simulink model "smueqq"  (R2017a)
settings: Solver=VariableStepAuto  StartTime=0.0  StopTime=180  RelTol=1e-3
libraries: dsparch4 x5, simulink x5, dspsnks4 x1, dspvision x1
settings Model: Creator=achar  LastModifiedBy=achar

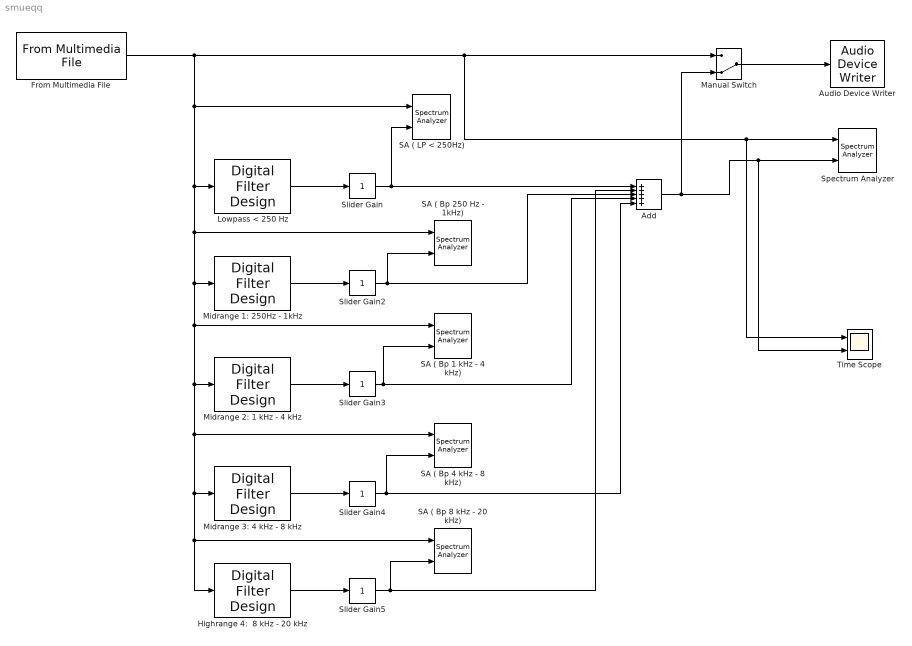
== system smueqq ==
  " Lowpass < 250 Hz " : dsparch4/Digital Filter Design  mwdsp_browser_bugfix_var=off
  Add : Sum  Inputs=+++++
  Audio Device Writer : dspsnks4/Audio Device Writer  Driver=DirectSound  Device=Default  InheritSampleRate=on  SampleRate=44100  BitDepth=16-bit integer  BufferSize=4096  NumBuffers=10  DefaultOutputChannelMapping=on  OutputChannelMapping=1:2  OutputNumUnderrunSamples=off  DriverIdx=1  DeviceWarnFlag=''
  From Multimedia File : dspvision/From Multimedia File  inputFilename=D:\BitBucketLocalRepository\projects\digital_signal_processing\P1_5_band_Audio_Equalizer_Matlab\FIR_BASED\BE_OE.mp3  loop=on  numPlays=inf  outputStreams=Audio only  videoDataType=single  audioDataType=double  inheritSampleTime=on  userDefinedSampleTime=1/30  noAudioOutput=off  isIntensityVideo=off  fourcc=RGB  colorVideoFormat=Separate color signals  outputEOF=off  dataOrg=Column-major  audioFrameSize=1024  computeAudioFrameSize=off  outSamplingMode=Sample based
      settings: SourceProductBaseCode=VP
  Highrange 4:  8 kHz - 20 kHz : dsparch4/Digital Filter Design  mwdsp_browser_bugfix_var=off
  Manual Switch : ManualSwitch  CurrentSetting=0
  "Midrange 1: 250Hz - 1kHz " : dsparch4/Digital Filter Design  mwdsp_browser_bugfix_var=off
  Midrange 2: 1 kHz - 4 kHz : dsparch4/Digital Filter Design  mwdsp_browser_bugfix_var=off
  Midrange 3: 4 kHz - 8 kHz : dsparch4/Digital Filter Design  mwdsp_browser_bugfix_var=off
  SA ( Bp 1 kHz - 4 kHz) : SpectrumAnalyzer  NumInputPorts=2
  SA ( Bp 250 Hz - 1kHz) : SpectrumAnalyzer  NumInputPorts=2
  SA ( Bp 4 kHz - 8 kHz) : SpectrumAnalyzer  NumInputPorts=2
  SA ( Bp 8 kHz - 20 kHz) : SpectrumAnalyzer  NumInputPorts=2
  SA ( LP < 250Hz) : SpectrumAnalyzer  NumInputPorts=2
  Slider Gain{,2..5} (5 alike) : simulink/Math Operations/Slider Gain  gain=1  low=-15  high=15
  Spectrum Analyzer : SpectrumAnalyzer  NumInputPorts=2
  Time Scope : Scope  NumInputPorts=2
  wires:
  " Lowpass < 250 Hz "/1 -> Slider Gain/1
  Manual Switch/1 -> Audio Device Writer/1
  Add/1 -> Time Scope/2, Spectrum Analyzer/2, Manual Switch/2
  Slider Gain/1 -> SA ( LP < 250Hz)/2, Add/1
  "Midrange 1: 250Hz - 1kHz "/1 -> Slider Gain2/1
  Midrange 2: 1 kHz - 4 kHz/1 -> Slider Gain3/1
  Slider Gain2/1 -> SA ( Bp 250 Hz - 1kHz)/2, Add/3
  Slider Gain3/1 -> SA ( Bp 1 kHz - 4 kHz)/2, Add/4
  Midrange 3: 4 kHz - 8 kHz/1 -> Slider Gain4/1
  Slider Gain4/1 -> SA ( Bp 4 kHz - 8 kHz)/2, Add/5
  Highrange 4:  8 kHz - 20 kHz/1 -> Slider Gain5/1
  Slider Gain5/1 -> SA ( Bp 8 kHz - 20 kHz)/2, Add/2
  From Multimedia File/1 -> Time Scope/1, Spectrum Analyzer/1, Manual Switch/1, SA ( LP < 250Hz)/1, SA ( Bp 4 kHz - 8 kHz)/1, SA ( Bp 8 kHz - 20 kHz)/1, Highrange 4:  8 kHz - 20 kHz/1, Midrange 3: 4 kHz - 8 kHz/1, Midrange 2: 1 kHz - 4 kHz/1, SA ( Bp 1 kHz - 4 kHz)/1, "Midrange 1: 250Hz - 1kHz "/1, SA ( Bp 250 Hz - 1kHz)/1, " Lowpass < 250 Hz "/1
